simulink model "DistrictScreening"  (R2026a)
settings: Solver=FixedStepDiscrete  StopTime=arrivals(end,1)  FixedStep=1
undefined symbols (not defined in the file or in its folder): capAI, capCapture, capReview, capUploadMB, mbPerPatient, reviewFraction
settings Model: Creator=Manosh  LastModifiedBy=Manosh

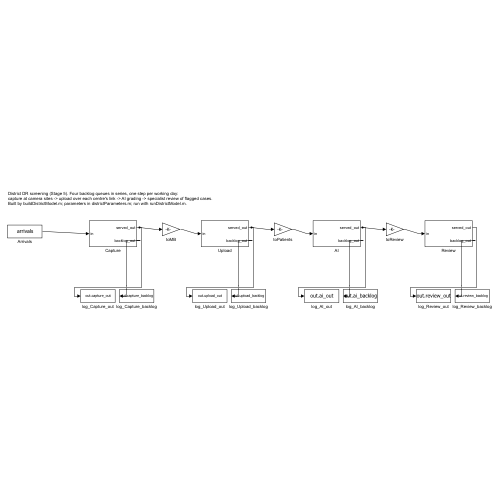
[thumbnail: Simulink's stored preview of the top-level diagram]
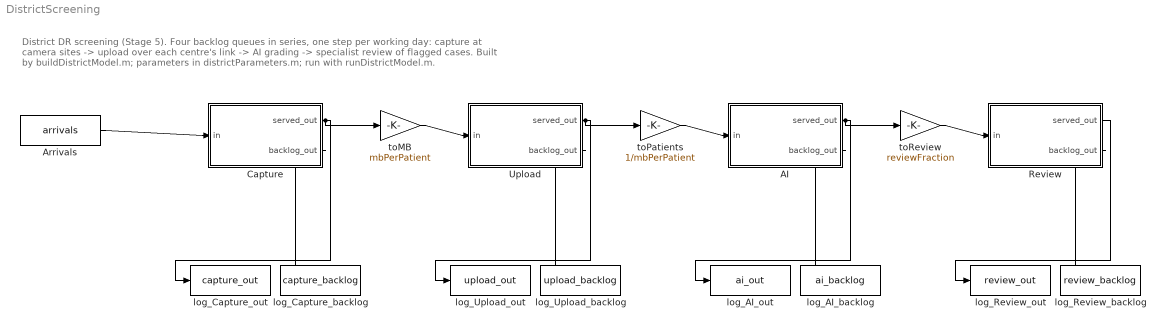
== system DistrictScreening ==
  note: District DR screening (Stage 5). Four backlog queues in series, one step per working day:
      | capture at camera sites -> upload over each centre's link -> AI grading -> specialist review of flagged cases.
      | Built by buildDistrictModel.m; parameters in districtParameters.m; run with runDistrictModel.m.
  AI : Subsystem
  Arrivals : FromWorkspace  VariableName=arrivals  SampleTime=1  Interpolate=off  OutputAfterFinalValue=Setting to zero
  Capture : Subsystem
  Review : Subsystem
  Upload : Subsystem
  log_AI_backlog : ToWorkspace  VariableName=ai_backlog  SampleTime=1
  log_AI_out : ToWorkspace  VariableName=ai_out  SampleTime=1
  log_Capture_backlog : ToWorkspace  VariableName=capture_backlog  SampleTime=1
  log_Capture_out : ToWorkspace  VariableName=capture_out  SampleTime=1
  log_Review_backlog : ToWorkspace  VariableName=review_backlog  SampleTime=1
  log_Review_out : ToWorkspace  VariableName=review_out  SampleTime=1
  log_Upload_backlog : ToWorkspace  VariableName=upload_backlog  SampleTime=1
  log_Upload_out : ToWorkspace  VariableName=upload_out  SampleTime=1
  toMB : Gain  Gain=mbPerPatient
  toPatients : Gain  Gain=1/mbPerPatient
  toReview : Gain  Gain=reviewFraction
  wires:
  Arrivals/1 -> Capture/1(in)
  Capture/1(served_out) -> toMB/1, log_Capture_out/1
  toMB/1 -> Upload/1(in)
  Upload/1(served_out) -> toPatients/1, log_Upload_out/1
  toPatients/1 -> AI/1(in)
  AI/1(served_out) -> toReview/1, log_AI_out/1
  toReview/1 -> Review/1(in)
  Capture/2(backlog_out) -> log_Capture_backlog/1
  Upload/2(backlog_out) -> log_Upload_backlog/1
  AI/2(backlog_out) -> log_AI_backlog/1
  Review/1(served_out) -> log_Review_out/1
  Review/2(backlog_out) -> log_Review_backlog/1

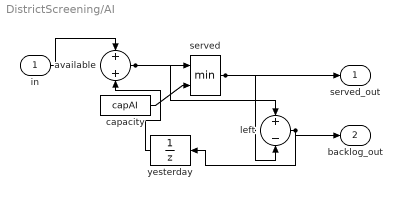
== system DistrictScreening/AI ==
  in : Inport
  available : Sum
  capacity : Constant  Value=capAI  SampleTime=1
  left : Sum  Inputs=+-
  served : MinMax  Inputs=2
  yesterday : UnitDelay
  served_out : Outport
  backlog_out : Outport  Port=2
  wires:
  in/1 -> available/1
  yesterday/1 -> available/2
  available/1 -> served/1, left/1
  capacity/1 -> served/2
  served/1 -> left/2, served_out/1
  left/1 -> backlog_out/1, yesterday/1

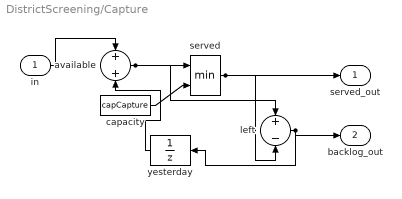
== system DistrictScreening/Capture ==
  in : Inport
  available : Sum
  capacity : Constant  Value=capCapture  SampleTime=1
  left : Sum  Inputs=+-
  served : MinMax  Inputs=2
  yesterday : UnitDelay
  served_out : Outport
  backlog_out : Outport  Port=2
  wires:
  in/1 -> available/1
  yesterday/1 -> available/2
  available/1 -> served/1, left/1
  capacity/1 -> served/2
  served/1 -> left/2, served_out/1
  left/1 -> backlog_out/1, yesterday/1

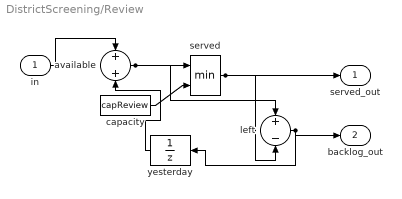
== system DistrictScreening/Review ==
  in : Inport
  available : Sum
  capacity : Constant  Value=capReview  SampleTime=1
  left : Sum  Inputs=+-
  served : MinMax  Inputs=2
  yesterday : UnitDelay
  served_out : Outport
  backlog_out : Outport  Port=2
  wires:
  in/1 -> available/1
  yesterday/1 -> available/2
  available/1 -> served/1, left/1
  capacity/1 -> served/2
  served/1 -> left/2, served_out/1
  left/1 -> backlog_out/1, yesterday/1

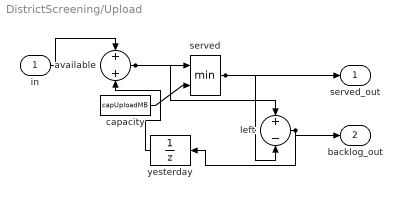
== system DistrictScreening/Upload ==
  in : Inport
  available : Sum
  capacity : Constant  Value=capUploadMB  SampleTime=1
  left : Sum  Inputs=+-
  served : MinMax  Inputs=2
  yesterday : UnitDelay
  served_out : Outport
  backlog_out : Outport  Port=2
  wires:
  in/1 -> available/1
  yesterday/1 -> available/2
  available/1 -> served/1, left/1
  capacity/1 -> served/2
  served/1 -> left/2, served_out/1
  left/1 -> backlog_out/1, yesterday/1
